simulink model "prep_real"  (R2023b)
settings: Solver=ode45  StartTime=0.0  StopTime=2200  RelTol=1e-3  EnableMultiTasking=on
undefined symbols (not defined in the file or in its folder): Advantech, PCI
libraries: sldrtlib x4
settings Model: Creator=Admin  LastModifiedBy=andre
settings SolverCC: AlgebraicLoopSolver=TrustRegion
settings DataIOCC: LimitDataPoints=on  SaveFormat=Array  ReturnWorkspaceOutputs=off
settings OptimizationCC: ReuseModelBlockBuffer=off  LifeSpan=inf
settings DebuggingCC: UnconnectedInputMsg=warning  UnconnectedOutputMsg=warning  UnconnectedLineMsg=warning  SFUnexpectedBacktrackingDiag=warning  SFNoUnconditionalDefaultTransitionDiag=warning  SFExecutionAtInitializationDiag=none  ArithmeticOperatorsInVariantConditions=warning
settings HardwareCC: ProdBitPerPointer=32  ProdBitPerSizeT=32  ProdBitPerPtrDiffT=32  ProdLargestAtomicFloat=None  ProdIntDivRoundTo=Undefined  ProdEndianess=Unspecified  ProdWordSize=32  ProdHWDeviceType=32-bit Generic
settings ModelReferenceCC: PropagateSignalLabelsOutOfModel=off
settings SFSimCC: SimUseLocalCustomCode=off  CustomCodeUndefinedFunction=UseInterfaceOnly
settings RTWCC: RTWUseLocalCustomCode=off
settings CodeAppCC: StateflowObjectComments=on
settings GRTTargetCC: TargetLangStandard=C89/C90 (ANSI)
settings ConfigComp: CovMetricSettings=dw  CovSaveCumulativeToWorkspaceVar=on  CovSaveSingleToWorkspaceVar=on  CovExternalEMLEnable=off

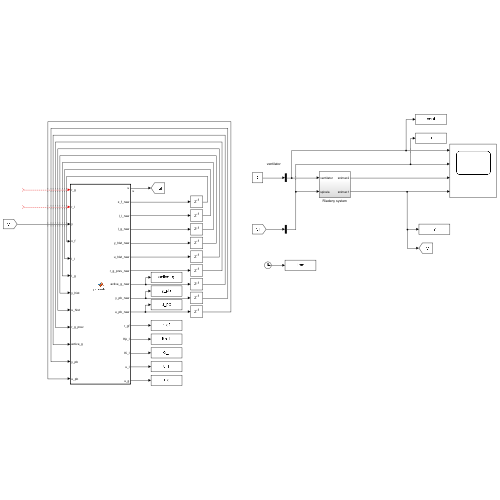
[thumbnail: Simulink's stored preview of the top-level diagram]
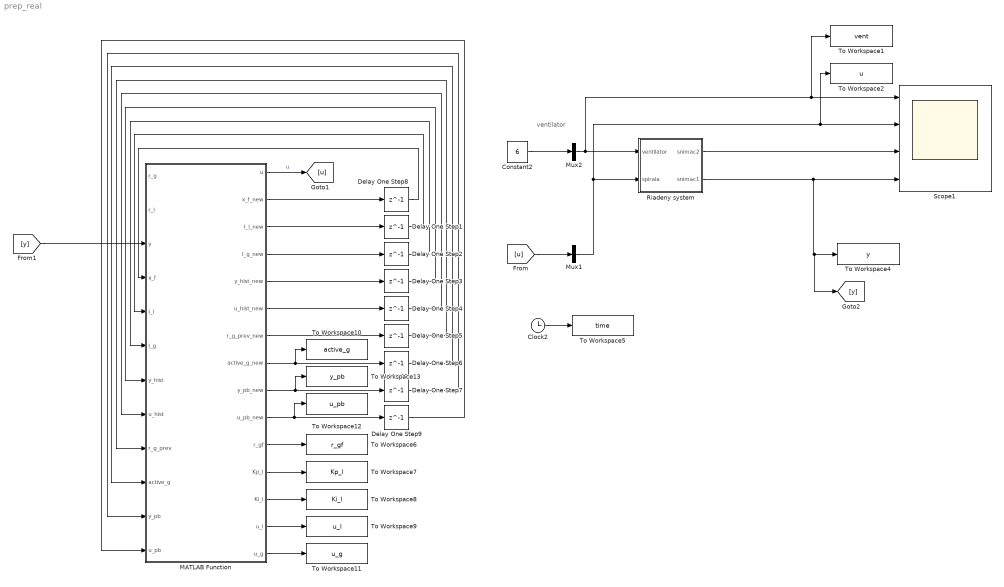
== system prep_real ==
  note: ventilator
  Clock2 : Clock
  Constant2 : Constant  Value=6
  Delay One Step{1..9} (9 alike) : Delay  DelayLength=1
  MATLAB Function : MATLAB Function  TreatAsAtomicUnit=on
  Mux1 : Mux  Inputs=1
  Mux2 : Mux  Inputs=1
  Riadeny system : Subsystem
  Scope1 : Scope  NumInputPorts=4
  To Workspace1 : ToWorkspace  VariableName=vent  SampleTime=0.1
      settings: Save2DSignal=2-D array (concatenate along first dimension)
  To Workspace10 : ToWorkspace  VariableName=active_g  SampleTime=0.1
      settings: Save2DSignal=2-D array (concatenate along first dimension)
  To Workspace11 : ToWorkspace  VariableName=u_g  SampleTime=0.1
      settings: Save2DSignal=2-D array (concatenate along first dimension)
  To Workspace12 : ToWorkspace  VariableName=u_pb  SampleTime=0.1
      settings: Save2DSignal=2-D array (concatenate along first dimension)
  To Workspace13 : ToWorkspace  VariableName=y_pb  SampleTime=0.1
      settings: Save2DSignal=2-D array (concatenate along first dimension)
  To Workspace2 : ToWorkspace  VariableName=u  SampleTime=0.1
      settings: Save2DSignal=2-D array (concatenate along first dimension)
  To Workspace4 : ToWorkspace  VariableName=y  SampleTime=0.1
      settings: Save2DSignal=2-D array (concatenate along first dimension)
  To Workspace5 : ToWorkspace  VariableName=time  SampleTime=0.1
      settings: Save2DSignal=2-D array (concatenate along first dimension)
  To Workspace6 : ToWorkspace  VariableName=r_gf  SampleTime=0.1
      settings: Save2DSignal=2-D array (concatenate along first dimension)
  To Workspace7 : ToWorkspace  VariableName=Kp_l  SampleTime=0.1
      settings: Save2DSignal=2-D array (concatenate along first dimension)
  To Workspace8 : ToWorkspace  VariableName=Ki_l  SampleTime=0.1
      settings: Save2DSignal=2-D array (concatenate along first dimension)
  To Workspace9 : ToWorkspace  VariableName=u_l  SampleTime=0.1
      settings: Save2DSignal=2-D array (concatenate along first dimension)
  wires:
  Mux2/1 -> Riadeny system/1(ventilator), To Workspace1/1, Scope1/1
  Riadeny system/1(snimac2) -> Scope1/3
  Riadeny system/2(snimac1) -> [y], To Workspace4/1, Scope1/4
  Mux1/1 -> Riadeny system/2(spirala), To Workspace2/1, Scope1/2
  Constant2/1 -> Mux2/1
  [u] -> Mux1/1
  Clock2/1 -> To Workspace5/1
  MATLAB Function/13(Ki_l) -> To Workspace8/1
  MATLAB Function/12(Kp_l) -> To Workspace7/1
  MATLAB Function/14(u_l) -> To Workspace9/1
  MATLAB Function/10(u_pb_new) -> To Workspace12/1, Delay One Step9/1
  MATLAB Function/7(r_g_prev_new) -> Delay One Step5/1
  MATLAB Function/6(u_hist_new) -> Delay One Step4/1
  MATLAB Function/3(I_l_new) -> Delay One Step1/1
  MATLAB Function/5(y_hist_new) -> Delay One Step3/1
  ? -> MATLAB Function/2(r_l)
  Delay One Step7/1 -> MATLAB Function/11(y_pb)
  [y] -> MATLAB Function/3(y)
  Delay One Step5/1 -> MATLAB Function/9(r_g_prev)
  Delay One Step3/1 -> MATLAB Function/7(y_hist)
  MATLAB Function/9(y_pb_new) -> To Workspace13/1, Delay One Step7/1
  MATLAB Function/2(x_f_new) -> Delay One Step8/1
  Delay One Step8/1 -> MATLAB Function/4(x_f)
  Delay One Step4/1 -> MATLAB Function/8(u_hist)
  Delay One Step2/1 -> MATLAB Function/6(I_g)
  MATLAB Function/4(I_g_new) -> Delay One Step2/1
  Delay One Step6/1 -> MATLAB Function/10(active_g)
  Delay One Step9/1 -> MATLAB Function/12(u_pb)
  MATLAB Function/8(active_g_new) -> To Workspace10/1, Delay One Step6/1
  MATLAB Function/15(u_g) -> To Workspace11/1
  ? -> MATLAB Function/1(r_g)
  Delay One Step1/1 -> MATLAB Function/5(I_l)
  MATLAB Function/11(r_gf) -> To Workspace6/1
  MATLAB Function/1(u) -> [u]  "u"

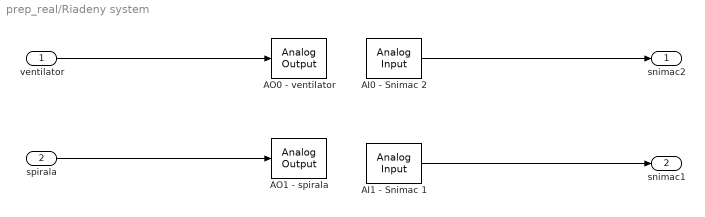
== system prep_real/Riadeny system ==
  ventilator : Inport
  spirala : Inport  Port=2
  AI0 - Snimac 2 : sldrtlib/Analog Input  SampleTime=0.1  MaxMissedTicks=10  ShowMissedTicks=off  YieldWhenWaiting=off  DrvName=Advantech/PCI-1711  DrvAddress=4294967295  DrvOptions=zeros(1,0)  Channels=1  RangeMode=1  VoltRange=1  DataType=1
      settings: AttributesFormatString=Advantech\nPCI-1711 [auto]
  AI1 - Snimac 1 : sldrtlib/Analog Input  SampleTime=0.1  MaxMissedTicks=10  ShowMissedTicks=off  YieldWhenWaiting=off  DrvName=Advantech/PCI-1711  DrvAddress=4294967295  DrvOptions=zeros(1,0)  Channels=2  RangeMode=1  VoltRange=1  DataType=1
      settings: AttributesFormatString=Advantech\nPCI-1711 [auto]
  AO0 - ventilator : sldrtlib/Analog Output  SampleTime=0.1  MaxMissedTicks=10  ShowMissedTicks=off  YieldWhenWaiting=off  DrvName=Advantech/PCI-1711  DrvAddress=4294967295  DrvOptions=zeros(1,0)  Channels=1  RangeMode=1  VoltRange=2  InitialValue=[]  FinalValue=[]
      settings: AttributesFormatString=Advantech\nPCI-1711 [auto]
  AO1 - spirala : sldrtlib/Analog Output  SampleTime=0.1  MaxMissedTicks=10  ShowMissedTicks=off  YieldWhenWaiting=off  DrvName=Advantech/PCI-1711  DrvAddress=4294967295  DrvOptions=zeros(1,0)  Channels=2  RangeMode=1  VoltRange=2  InitialValue=[]  FinalValue=[]
      settings: AttributesFormatString=Advantech\nPCI-1711 [auto]
  snimac2 : Outport
  snimac1 : Outport  Port=2
  wires:
  ventilator/1 -> AO0 - ventilator/1
  spirala/1 -> AO1 - spirala/1
  AI1 - Snimac 1/1 -> snimac1/1
  AI0 - Snimac 2/1 -> snimac2/1

== matlab function prep_real/MATLAB Function ==
  data: r_g input size=[1 1]; r_l input size=[1 1]; y input size=[1 1]; u output size=[1 1]; x_f_new output size=[2 1]; I_l_new output size=[1 1]; x_f input size=[2 1]; I_g_new output size=[1 1]; I_l input size=[1 1]; I_g input size=[1 1]; y_hist input size=[30 1]; y_hist_new output size=[30 1]; u_hist_new output size=[30 1]; r_g_prev_new output size=[1 1]; active_g_new output size=[1 1]; u_hist input size=[30 1]; r_g_prev input size=[1 1]; active_g input size=[1 1]; y_pb_new output size=[1 1]; u_pb_new output size=[1 1]; y_pb input size=[1 1]; u_pb input size=[1 1]; r_gf output; Kp_l output; Ki_l output; u_l output; u_g output
function [u, x_f_new, I_l_new, I_g_new, y_hist_new, u_hist_new, ...
          r_g_prev_new, active_g_new, y_pb_new, u_pb_new, r_gf, Kp_l, Ki_l, u_l, u_g] = ...
          pi_switch(r_g, r_l, y, x_f, I_l, I_g, y_hist, u_hist, ...
          r_g_prev, active_g, y_pb, u_pb)

Ts = 0.1;

%Global PI
Kp_g = 1;
Ki_g = 0.1;

%Gain sced table
y_pb_table = [4.4884; 6.3412; 7.7441];
u_pb_table = [2; 4; 6];
Kp_l_table = [2.77; 3.58; 1.83];
Ki_l_table = [1.48; 1.84; 2.2];

%filter matrices
A_f = [0, 1
       -0.01, -0.2];

b_f = [0;
       1];

c_f = [0.01, 0];

% 1 Detect step change
if r_g ~= r_g_prev
    active_g = 1;
end

% 2 Filter global reference
r_gf = c_f * x_f;
x_f_new = x_f + (A_f * x_f + b_f * r_g)*Ts;

% 3 Select local points PI params
dist_pb = abs(y_pb_table - y_pb);
[~, idx_pb] = min(dist_pb);

Kp_l = Kp_l_table(idx_pb);
Ki_l = Ki_l_table(idx_pb);

% 4 Control errors
e_l = r_l - (y - y_pb);
e_g = r_gf - y;

% 5 Control law
u_l = (1 - active_g) * (u_pb + Kp_l * e_l + Ki_l * I_l);
u_g = active_g * (Kp_g * e_g + Ki_g * I_g);
u = u_l + u_g;

% 6 Update histories
y_hist_new = [y_hist(2:end); y];
u_hist_new = [u_hist(2:end); u];

% 7 Setting detection
lower_bound = r_g - 0.7 * r_g;
upper_bound = r_g + 0.7 * r_g;

count_ok = 0;
for i = 1:30
    if (y_hist_new(i) >= lower_bound) && (y_hist_new(i) <= upper_bound)
        count_ok = count_ok + 1;
    end
end

y_pb_new = y_pb;
u_pb_new = u_pb;
active_g_new = active_g;

if active_g == 1 && count_ok >= 25
    y_pb_est = mean(y_hist_new);
    u_pb_est = mean(u_hist_new);

    y_pb_new = y_pb_est;
    u_pb_new = u_pb_est;

    active_g_new = 0;
end

active_l = 1 - active_g;
active_l_new = 1 - active_g_new;

% 8 Integral states update
if active_l == 1
    I_l_new = I_l + e_l * Ts;
else
    I_l_new = 0;  %((u - u_pb) - Kp_l * e_l) / Ki_l;
end

if active_g == 1
    I_g_new = I_g + e_g * Ts;
else
    I_g_new = (u - Kp_g * e_g) / Ki_g;
end

% % 9 Tracking for next step after switching
% if active_l_new == 1 && active_l == 0
%     dist_new = abs(y_pb_table - y_pb_new);
%     [~, idx_new] = min(dist_new);
% 
%     Kp_l_new = Kp_l_table(idx_new);
%     Ki_l_new = Ki_l_table(idx_new);
% 
%     e_l_new = r_l - (y - y_pb_new);
%     I_l_new = ((u - u_pb_new) - Kp_l_new * e_l_new) / Ki_l_new;
% end

% 10 memory update
r_g_prev_new = r_g;
